simulink model "quadcopter_plant_only"  (R2019b)
settings: Solver=VariableStepAuto  StartTime=0.0  StopTime=10.0  RelTol=1e-3
undefined symbols (not defined in the file or in its folder): param
libraries: vrlib x2
settings Model: Creator=emiel  LastModifiedBy=emiel

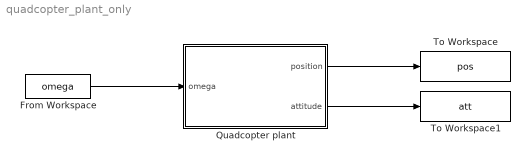
== system quadcopter_plant_only ==
  From Workspace : FromWorkspace  VariableName=omega  SampleTime=0
  Quadcopter plant : Subsystem
  To Workspace : ToWorkspace  VariableName=pos  SaveFormat=Timeseries  SampleTime=-1
  To Workspace1 : ToWorkspace  VariableName=att  SaveFormat=Timeseries  SampleTime=-1
  wires:
  From Workspace/1 -> Quadcopter plant/1(omega)
  Quadcopter plant/1(position) -> To Workspace/1
  Quadcopter plant/2(attitude) -> To Workspace1/1

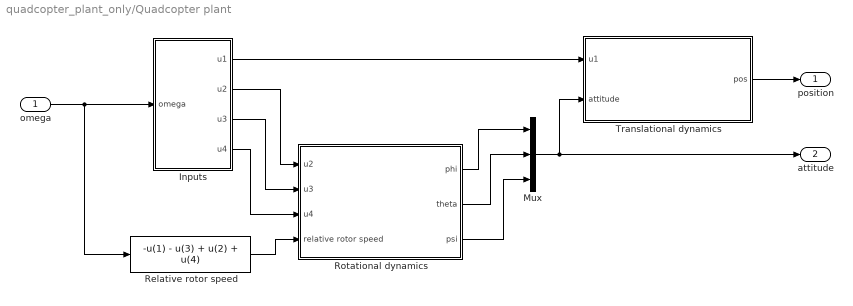
== system quadcopter_plant_only/Quadcopter plant ==
  omega : Inport
  Inputs : Subsystem
  Mux : Mux  Inputs=3
  Relative rotor speed : Fcn  Expr=-u(1) - u(3) + u(2) + u(4)
  Rotational dynamics : Subsystem
  Translational dynamics : Subsystem
  position : Outport
  attitude : Outport  Port=2
  wires:
  Mux/1 -> Translational dynamics/2(attitude), attitude/1
  omega/1 -> Relative rotor speed/1, Inputs/1(omega)
  Inputs/2(u2) -> Rotational dynamics/1(u2)
  Rotational dynamics/1(phi) -> Mux/1
  Relative rotor speed/1 -> Rotational dynamics/4(relative rotor speed)
  Inputs/3(u3) -> Rotational dynamics/2(u3)
  Inputs/4(u4) -> Rotational dynamics/3(u4)
  Inputs/1(u1) -> Translational dynamics/1(u1)
  Rotational dynamics/2(theta) -> Mux/2
  Rotational dynamics/3(psi) -> Mux/3
  Translational dynamics/1(pos) -> position/1

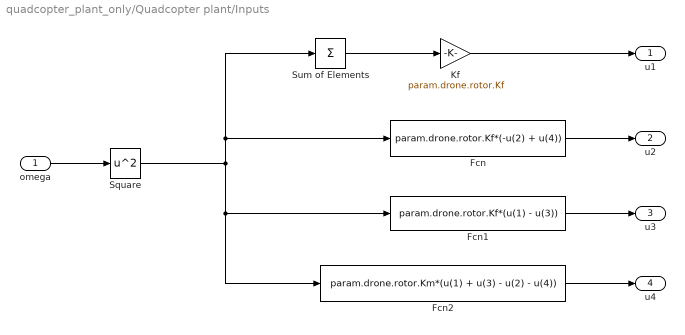
== system quadcopter_plant_only/Quadcopter plant/Inputs ==
  omega : Inport
  Fcn : Fcn  Expr=param.drone.rotor.Kf*(-u(2) + u(4))
  Fcn1 : Fcn  Expr=param.drone.rotor.Kf*(u(1) - u(3))
  Fcn2 : Fcn  Expr=param.drone.rotor.Km*(u(1) + u(3) - u(2) - u(4))
  Kf : Gain  Gain=param.drone.rotor.Kf
  Square : Math  Operator=square  SignedPower=off  SaturateOnIntegerOverflow=on
  Sum of Elements : Sum  Inputs=+
  u1 : Outport
  u2 : Outport  Port=2
  u3 : Outport  Port=3
  u4 : Outport  Port=4
  wires:
  omega/1 -> Square/1
  Sum of Elements/1 -> Kf/1
  Kf/1 -> u1/1
  Square/1 -> Fcn2/1, Fcn1/1, Sum of Elements/1, Fcn/1
  Fcn1/1 -> u3/1
  Fcn/1 -> u2/1
  Fcn2/1 -> u4/1

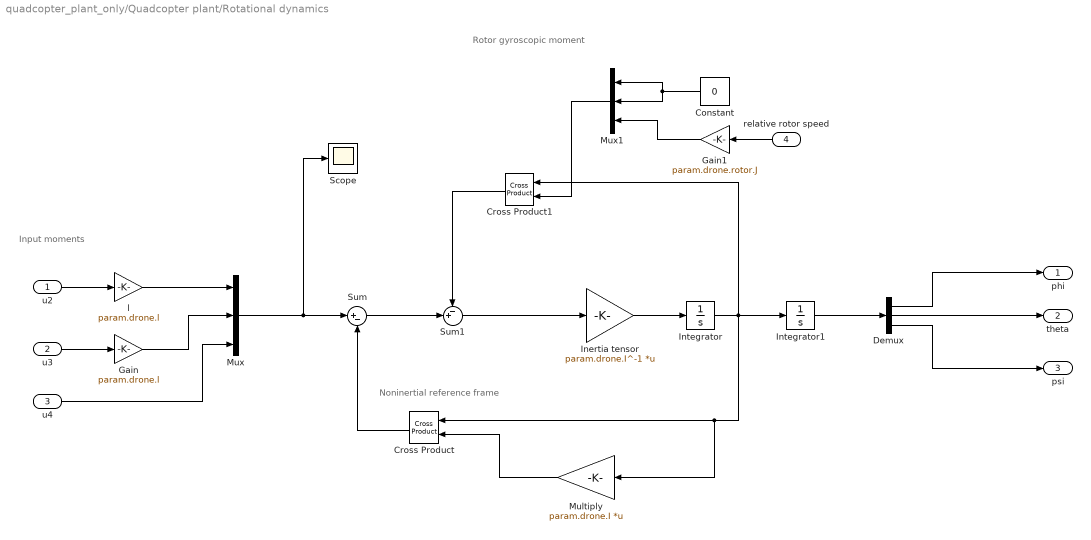
== system quadcopter_plant_only/Quadcopter plant/Rotational dynamics ==
  note: Input moments
  note: Noninertial reference frame
  note: Rotor gyroscopic moment
  u2 : Inport
  u3 : Inport  Port=2
  u4 : Inport  Port=3
  relative rotor speed : Inport  Port=4
  Constant : Constant  Value=0
  Cross Product : vrlib/Utilities/Cross Product
      settings: SourceProductName=Simulink
  Cross Product1 : vrlib/Utilities/Cross Product
      settings: SourceProductName=Simulink
  Demux : Demux  Outputs=3
  Gain : Gain  Gain=param.drone.l
  Gain1 : Gain  Gain=param.drone.rotor.J
  Inertia tensor : Gain  Gain=param.drone.I^-1  Multiplication=Matrix(K*u) (u vector)
  Integrator : Integrator  InitialCondition=param.x0.angvel
  Integrator1 : Integrator  InitialCondition=param.x0.att
  Multiply : Gain  Gain=param.drone.I  Multiplication=Matrix(K*u) (u vector)
  Mux : Mux  Inputs=3
  Mux1 : Mux  Inputs=3
  Scope : Scope
  Sum : Sum  Inputs=|+-
  Sum1 : Sum  Inputs=-+|
  l : Gain  Gain=param.drone.l
  phi : Outport
  theta : Outport  Port=2
  psi : Outport  Port=3
  wires:
  Integrator1/1 -> Demux/1
  Demux/3 -> psi/1
  Demux/2 -> theta/1
  Demux/1 -> phi/1
  u2/1 -> l/1
  u3/1 -> Gain/1
  Inertia tensor/1 -> Integrator/1
  u4/1 -> Mux/3
  l/1 -> Mux/1
  Gain/1 -> Mux/2
  Mux/1 -> Scope/1, Sum/1
  Integrator/1 -> Cross Product1/1, Cross Product/1, Multiply/1, Integrator1/1
  Cross Product/1 -> Sum/2
  relative rotor speed/1 -> Gain1/1
  Constant/1 -> Mux1/2, Mux1/1
  Sum/1 -> Sum1/2
  Cross Product1/1 -> Sum1/1
  Mux1/1 -> Cross Product1/2
  Multiply/1 -> Cross Product/2
  Sum1/1 -> Inertia tensor/1
  Gain1/1 -> Mux1/3

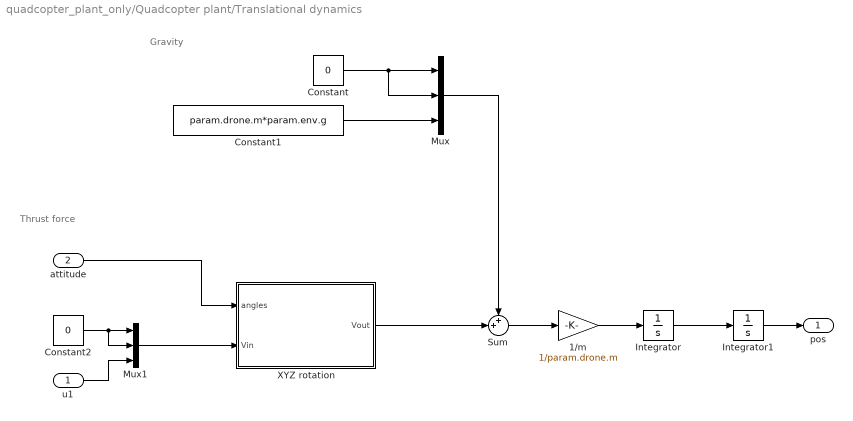
== system quadcopter_plant_only/Quadcopter plant/Translational dynamics ==
  note: Thrust force
  note: Gravity
  u1 : Inport
  attitude : Inport  Port=2
  1/m : Gain  Gain=1/param.drone.m
  Constant : Constant  Value=0
  Constant1 : Constant  Value=param.drone.m*param.env.g
  Constant2 : Constant  Value=0
  Integrator : Integrator  InitialCondition=param.x0.linvel
  Integrator1 : Integrator  InitialCondition=param.x0.pos
  Mux : Mux  Inputs=3
  Mux1 : Mux  Inputs=3
  Sum : Sum  Inputs=++|
  XYZ rotation : MATLAB Function  TreatAsAtomicUnit=on
  pos : Outport
  wires:
  attitude/1 -> XYZ rotation/1(angles)
  Constant/1 -> Mux/2, Mux/1
  Constant1/1 -> Mux/3
  XYZ rotation/1(Vout) -> Sum/2
  Mux/1 -> Sum/1
  Sum/1 -> 1/m/1
  Integrator/1 -> Integrator1/1
  Integrator1/1 -> pos/1
  1/m/1 -> Integrator/1
  Constant2/1 -> Mux1/2, Mux1/1
  u1/1 -> Mux1/3
  Mux1/1 -> XYZ rotation/2(Vin)

== matlab function quadcopter_plant_only/Quadcopter plant/Translational dynamics/XYZ rotation ==
  data: angles input; Vout output; Vin input
function Vout = rotationXYZ(angles, Vin)
    R = eul2rotm(angles, 'XYZ');
    Vout = R*Vin;
